simulink model "WTP"  (R2020a)
settings: Solver=FixedStepAuto  StartTime=0.0  StopTime=200  FixedStep=1e-2  RelTol=1e-3
values from neighbouring files (symbols this model uses):
  alpha = 0.018    [ParetoWTP.mat]    (also in WTPInit.m; WTPOP.m; sfun_WTP.m = param(5))
  beta = 0.2    [ParetoWTP.mat]    (also in WTPInit.m; WTPOP.m; sfun_WTP.m = param(3))
  D0 = 0.025    [ParetoWTP.mat]    (also in WTPInit.m)
  DO0 = 5    [ParetoWTP.mat]    (also in WTPInit.m)
  DOin0 = 0.5    [ParetoWTP.mat]    (also in WTPInit.m)
  DOmax = 10    [ParetoWTP.mat]    (also in WTPInit.m; WTPOP.m; sfun_WTP.m = param(9))
  K0 = 0.5    [ParetoWTP.mat]    (also in WTPInit.m; WTPOP.m; sfun_WTP.m = param(8))
  KDO = 2    [ParetoWTP.mat]    (also in WTPInit.m; WTPOP.m; sfun_WTP.m = param(4))
  Ks = 100    [ParetoWTP.mat]    (also in WTPInit.m; WTPOP.m; sfun_WTP.m = param(7))
  Qair0 = 27.5735    [ParetoWTP.mat]    (also in WTPInit.m)
  r = 0.6    [ParetoWTP.mat]    (also in WTPInit.m; WTPOP.m; sfun_WTP.m = param(2))
  S0 = 10.2941    [ParetoWTP.mat]    (also in WTPInit.m)
  Sin0 = 200    [ParetoWTP.mat]    (also in WTPInit.m)
  umax = 0.15    [ParetoWTP.mat]    (also in WTPInit.m; WTPOP.m; sfun_WTP.m = param(6))
  X0 = 298.2353    [ParetoWTP.mat]    (also in WTPInit.m)
  Xr0 = 596.4706    [ParetoWTP.mat]    (also in WTPInit.m)
  Y = 0.65    [ParetoWTP.mat]    (also in WTPInit.m; WTPOP.m; sfun_WTP.m = param(1))
settings Model: Creator=david  LastModifiedBy=david

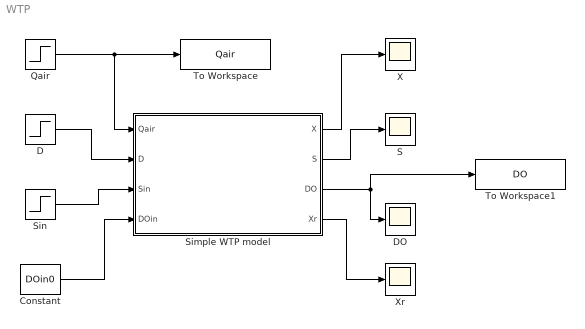
== system WTP ==
  Constant : Constant  Value=DOin0
  D : Step  Before=D0  After=D0  SampleTime=0
  DO : Scope
  Qair : Step  Time=100  Before=Qair0  After=Qair0*1.4  SampleTime=0
  S : Scope
  Simple WTP model : Subsystem  mask{Y=Y, r=r, beta=beta, KDO=KDO, alpha=alpha, umax=umax, Ks=Ks, K0=K0, DOmax=DOmax, X0=X0, S0=S0, DO0=DO0, Xr0=Xr0}
      mask prompts: Y "Y ="; r "r ="; beta "beta ="; KDO "KDO ="; alpha "alpha ="; umax "umax ="; Ks "Ks ="; K0 "K0 ="; DOmax "DOmax ="; X0 "X ="; S0 "S ="; DO0 "DO ="; Xr0 "Xr ="
      mask DialogControl DescGroupVar Prompt: Simple WTP
      mask DialogControl DescTextVar Prompt: Fourth order non-linear WTP model
      mask DialogControl Container3 Prompt: Initial state
      mask Display: image('WTPFigure.png'); % Use "Edit Image" on toolstrip to change.
  Sin : Step  Before=Sin0  After=Sin0  SampleTime=0
  To Workspace : ToWorkspace  VariableName=Qair  SaveFormat=Timeseries  SampleTime=1e-2
  To Workspace1 : ToWorkspace  VariableName=DO  SaveFormat=Timeseries  SampleTime=1e-2
  X : Scope
  Xr : Scope
  wires:
  Qair/1 -> Simple WTP model/1(Qair), To Workspace/1
  D/1 -> Simple WTP model/2(D)
  Sin/1 -> Simple WTP model/3(Sin)
  Constant/1 -> Simple WTP model/4(DOin)
  Simple WTP model/1(X) -> X/1
  Simple WTP model/2(S) -> S/1
  Simple WTP model/3(DO) -> To Workspace1/1, DO/1
  Simple WTP model/4(Xr) -> Xr/1

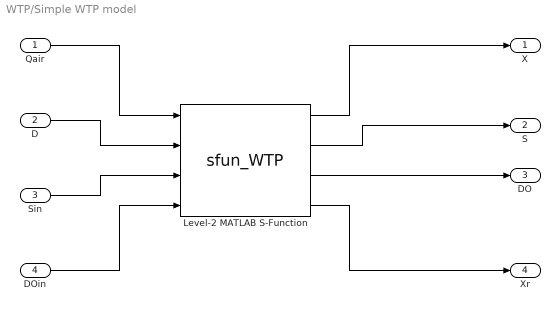
== system WTP/Simple WTP model ==
  Qair : Inport
  D : Inport  Port=2
  Sin : Inport  Port=3
  DOin : Inport  Port=4
  Level-2 MATLAB S-Function : M-S-Function  FunctionName=sfun_WTP  Parameters=|
      | [Y;
      | r;
      | beta;
      | KDO;alpha;
      | umax; Ks; K0;
      | DOmax], [X0;S0;DO0;Xr0]
  X : Outport
  S : Outport  Port=2
  DO : Outport  Port=3
  Xr : Outport  Port=4
  wires:
  Sin/1 -> Level-2 MATLAB S-Function/3
  Level-2 MATLAB S-Function/2 -> S/1
  Level-2 MATLAB S-Function/1 -> X/1
  Qair/1 -> Level-2 MATLAB S-Function/1
  D/1 -> Level-2 MATLAB S-Function/2
  Level-2 MATLAB S-Function/4 -> Xr/1
  DOin/1 -> Level-2 MATLAB S-Function/4
  Level-2 MATLAB S-Function/3 -> DO/1
